simulink model "VDCv2mk2"  (R2023b)
settings: Solver=FixedStepAuto  StartTime=0.0  StopTime=10.0  RelTol=1e-3
libraries: simulink x3
(part 2 of 2)

== system VDCv2mk2/SAFETY BLOCK/APPS_IMPLAUSIBILITY/Imp ==
  Action Port : ActionPort  ActionPortLabel=if(u1 > 0.1)
  Add : Sum
  Constant : Constant  OutDataTypeStr=boolean
  Data Store Read : DataStoreRead  DataStoreName=ERROR_Counter  IndexOptions=Index vector (dialog)  Indices=1  OutputSizes=1
  Out1 : Outport  VectorParamsAs1DForOutWhenUnconnected=off
  wires:
  Data Store Read/1 -> Add/1
  Constant/1 -> Add/2
  Add/1 -> Out1/1

== system VDCv2mk2/SAFETY BLOCK/APPS_IMPLAUSIBILITY/Not Imp ==
  Action Port : ActionPort  ActionPortLabel=else
  Constant : Constant  Value=0  OutDataTypeStr=double
  0 : Outport  VectorParamsAs1DForOutWhenUnconnected=off
  wires:
  Constant/1 -> 0/1  "Boolean"

== system VDCv2mk2/SAFETY BLOCK/APPS_IMPLAUSIBILITY/Signal_Failure ==
  Action Port : ActionPort  ActionPortLabel=if(u1>u2)
  Constant : Constant
  Out1 : Outport  VectorParamsAs1DForOutWhenUnconnected=off
  wires:
  Constant/1 -> Out1/1

== system VDCv2mk2/SAFETY BLOCK/APPS_IMPLAUSIBILITY/Signal_OK ==
  Action Port : ActionPort  ActionPortLabel=else
  Constant : Constant  Value=0
  Out1 : Outport  VectorParamsAs1DForOutWhenUnconnected=off
  wires:
  Constant/1 -> Out1/1

== system VDCv2mk2/Accumulator Power/PowerLimitDetection/OK_OrLatch/Latched Error ==
  Action Port : ActionPort  ActionPortLabel=if((u1>0))
  Constant : Constant
  "Out " : Outport  VectorParamsAs1DForOutWhenUnconnected=off
  wires:
  Constant/1 -> "Out "/1

== system VDCv2mk2/Accumulator Power/PowerLimitDetection/OK_OrLatch/OK ==
  Action Port : ActionPort  ActionPortLabel=else
  Constant : Constant  Value=0
  "Out " : Outport  VectorParamsAs1DForOutWhenUnconnected=off
  wires:
  Constant/1 -> "Out "/1

== matlab function VDCv2mk2/Brake_Light ==
  data: BP input; RM input; BL output; PS input; BL_threshold input
function BL = Brake_Light(BP, RM, PS, BL_threshold)
% PS = 0 -> braking
% PS = 1 -> lift
% PS = 2 -> accelerating
% BL_threshold -> BrakePedal percentage to activate BrakeLight
    if ((RM == 5 && PS == 0) || (RM ~= 5 && BP > BL_threshold))
        BL = 1;
        return;
    else
        BL = 0;
        return;
    end
end

== matlab function VDCv2mk2/ACCELERATION/RIGIDAXLE/Rigid Axle 2024  ==
  data: Throttle_Torque input; Motor_Torque_RR output; Motor_Torque_RL output
function [Motor_Torque_RR, Motor_Torque_RL] = RigidAxle_2024(Throttle_Torque)
    
    Motor_Torque_RR = Throttle_Torque;
    Motor_Torque_RL = Throttle_Torque;

end

== matlab function VDCv2mk2/ACCELERATION/RIGIDAXLE WITH TC/Rigid Axle with TC 2024  ==
  data: MAX_SLR input; Throttle_Torque input; Motor_Torque_RR output; Motor_Torque_RL output; el_Vel_X input; Max_Vel_ms_Wheel input
function [Motor_Torque_RR, Motor_Torque_RL] = RigidAxle_TC_2024(MAX_SLR, Throttle_Torque, el_Vel_X, Max_Vel_ms_Wheel)
if (el_Vel_X < 3 || Vel_ms_wheel_RR < 3 || Vel_ms_wheel_RL < 3)
    Motor_Torque_RR = Throttle_Torque_R;
    Motor_Torque_RL = Throttle_Torque_L;
    return;
else
    persistent correction
    if isempty(correction)
        correction = 0;
    end
% SLIP RATIO CALCULATIONS
    % calculate slip ratio
    if(el_Vel_X == 0 ||Max_Vel_ms_Wheel == 0)
        SLR = 1;
    else
    SLR = (Max_Vel_ms_Wheel / el_Vel_X);
    end
% CHECK FOR EXCESIVE SLIPPING
    % SLIP RATIO LESSER THAN MAXIMUM SLIP RATIO => apply max torque times throttle factor
        if(SLR < MAX_SLR)
            Motor_Torque_RR = Throttle_Torque; 
            Motor_Torque_RL = Throttle_Torque;
            correction = 0; %set correction to 0 as tyre is not slipping
            return;
        else
        % TYRE SLIPPING => TC INTERVENES
            % LOOK FOR THE PREVIOUS CORRECTION [Nm]
            if (correction == 0) % NOT SLIPPING PREVIOUSLY
                correction = 1; % [INTERVAL TO BE DETERMINED] set the correction to the torque we want to substract
                Motor_Torque_RR = Throttle_Torque - (1/33*correction^2+1/33*correction); % substract the correction from the torque to apply
                Motor_Torque_RL = Throttle_Torque - (1/33*correction^2+1/33*correction);
                return;
            else % TYRE SLIPPING PREVIOUSLY
                correction = correction + 1; % [INTERVAL TO BE DETERMINED] set the correction to the torque we want to substract + previous corrections
                Motor_Torque_RR = Throttle_Torque - (1/33*correction^2+1/33*correction); % substract the correction from the torque to apply
                Motor_Torque_RL = Throttle_Torque - (1/33*correction^2+1/33*correction);
                return;
            end
        end
end
end

== matlab function VDCv2mk2/ENDURANCE/RIGIDAXLE WITH TC/Rigid Axle with TC 2024  ==
  data: MAX_SLR input; Throttle_Torque input; Motor_Torque_RR output; Motor_Torque_RL output; el_Vel_X input; Max_Vel_ms_Wheel input
function [Motor_Torque_RR, Motor_Torque_RL] = RigidAxle_TC_2024(MAX_SLR, Throttle_Torque, el_Vel_X, Max_Vel_ms_Wheel)
if (el_Vel_X < 3 || Vel_ms_wheel_RR < 3 || Vel_ms_wheel_RL < 3)
    Motor_Torque_RR = Throttle_Torque_R;
    Motor_Torque_RL = Throttle_Torque_L;
    return;
else
    persistent correction
    if isempty(correction)
        correction = 0;
    end
% SLIP RATIO CALCULATIONS
    % calculate slip ratio
    if(el_Vel_X == 0 ||Max_Vel_ms_Wheel == 0)
        SLR = 1;
    else
    SLR = (Max_Vel_ms_Wheel / el_Vel_X);
    end
% CHECK FOR EXCESIVE SLIPPING
    % SLIP RATIO LESSER THAN MAXIMUM SLIP RATIO => apply max torque times throttle factor
        if(SLR < MAX_SLR)
            Motor_Torque_RR = Throttle_Torque; 
            Motor_Torque_RL = Throttle_Torque;
            correction = 0; %set correction to 0 as tyre is not slipping
            return;
        else
        % TYRE SLIPPING => TC INTERVENES
            % LOOK FOR THE PREVIOUS CORRECTION [Nm]
            if (correction == 0) % NOT SLIPPING PREVIOUSLY
                correction = 1; % [INTERVAL TO BE DETERMINED] set the correction to the torque we want to substract
                Motor_Torque_RR = Throttle_Torque - (1/33*correction^2+1/33*correction); % substract the correction from the torque to apply
                Motor_Torque_RL = Throttle_Torque - (1/33*correction^2+1/33*correction);
                return;
            else % TYRE SLIPPING PREVIOUSLY
                correction = correction + 1; % [INTERVAL TO BE DETERMINED] set the correction to the torque we want to substract + previous corrections
                Motor_Torque_RR = Throttle_Torque - (1/33*correction^2+1/33*correction); % substract the correction from the torque to apply
                Motor_Torque_RL = Throttle_Torque - (1/33*correction^2+1/33*correction);
                return;
            end
        end
end
end

== matlab function VDCv2mk2/ENDURANCE/TC+TV/MATLAB Function ==
  data: steering_max_angle input; Torque_R_Nm output; Torque_L_Nm output; steering input; steering_deadzone input; Throttle_Torque input; regen_en input; cg_slip input
function [Torque_R_Nm, Torque_L_Nm] = TV(steering_max_angle, steering, steering_deadzone, Throttle_Torque, regen_en, cg_slip)

if abs(steering) <= steering_deadzone % add steering deadzone (º)
    Torque_L_Nm = Throttle_Torque;
    Torque_R_Nm = Throttle_Torque;
    return;
end
if(abs(cg_slip) > (6*pi/180)) % check for driver correcting oversteer to avoid overcorrecting
     Torque_L_Nm = Throttle_Torque;
     Torque_R_Nm = Throttle_Torque;
     return;
end
d = (abs(steering) - steering_deadzone)/(steering_max_angle - steering_deadzone) * Throttle_Torque; %evaluate delta torque for given steering angle

if regen_en == 0 && d > Throttle_Torque
     d = Throttle_Torque; %force torque to be positive to avoid balance issues
end
if steering < -steering_deadzone %if steering left, apply full torque to the emotor on the outside
       %and substract the delta from the inside one
    Torque_L_Nm = Throttle_Torque-d;
    Torque_R_Nm = Throttle_Torque;
    return;
else
%opposite case
Torque_L_Nm = Throttle_Torque;
Torque_R_Nm = Throttle_Torque-d;
return;
end
end

== matlab function VDCv2mk2/ENDURANCE/TC+TV/TC 2024 ==
  data: MAX_SLR input; Throttle_Torque_R input; Throttle_Torque_L input; Motor_Torque_RR output; Motor_Torque_RL output; el_Vel_X input; Vel_ms_wheel_RR input; Vel_ms_wheel_RL input
function [Motor_Torque_RR, Motor_Torque_RL] = TC_2024(MAX_SLR,Throttle_Torque_R, Throttle_Torque_L, el_Vel_X, Vel_ms_wheel_RR, Vel_ms_wheel_RL)
if (el_Vel_X < 3 || Vel_ms_wheel_RR < 3 || Vel_ms_wheel_RL < 3)
    Motor_Torque_RR = Throttle_Torque_R;
    Motor_Torque_RL = Throttle_Torque_L;
    return;
else
    persistent correction
    if isempty(correction)
        correction = 0;
    end

% SLIP RATIO CALCULATIONS
    % calculate slip ratio
    if(el_Vel_X == 0 || Vel_ms_wheel_RR == 0)
        SLR_RR = 1;
    else
    SLR_RR = (Vel_ms_wheel_RR / el_Vel_X);
    end
    if(el_Vel_X == 0 || Vel_ms_wheel_RL == 0)
        SLR_RL = 1;
    else
    SLR_RL = (Vel_ms_wheel_RL / el_Vel_X);
    end


% SLIP RATIO CALCULATIONS
    % calculate slip ratio
    SLR = max(SLR_RR, SLR_RL);

% CHECK FOR EXCESIVE SLIPPING
    % SLIP RATIO LESSER THAN MAXIMUM SLIP RATIO => apply max torque times throttle factor
        if(SLR < MAX_SLR)
            Motor_Torque_RR = Throttle_Torque_R; 
            Motor_Torque_RL = Throttle_Torque_L;
            correction = 0; %set correction to 0 as tyre is not slipping
            return;
        else
        % TYRE SLIPPING => TC INTERVENES
            % LOOK FOR THE PREVIOUS CORRECTION [Nm]
            if (correction == 0) % NOT SLIPPING PREVIOUSLY
                correction = 1; % [INTERVAL TO BE DETERMINED] set the correction to the torque we want to substract
                Motor_Torque_RR = Throttle_Torque_R - (1/33*correction^2+1/33*correction); % substract the correction from the torque to apply
                Motor_Torque_RL = Throttle_Torque_L - (1/33*correction^2+1/33*correction);
                return;
            else % TYRE SLIPPING PREVIOUSLY
                correction = correction + 1; % [INTERVAL TO BE DETERMINED] set the correction to the torque we want to substract + previous corrections
                Motor_Torque_RR = Throttle_Torque_R - (1/33*correction^2+1/33*correction); % substract the correction from the torque to apply
                Motor_Torque_RL = Throttle_Torque_L - (1/33*correction^2+1/33*correction);
                return;
            end
        end
end
end

== matlab function VDCv2mk2/ACCELERATION/Torque demanded by the driver ==
  data: Throttle_Torque output; AP input; pedal_sat_down input; pedal_sat_up input; max_torque input
function Throttle_Torque  = TT(AP, pedal_sat_down, pedal_sat_up, max_torque)
    if AP <= pedal_sat_down %establish the lower deadzone for the throttle pedal
        Throttle_Response = 0;

    elseif AP >= pedal_sat_up %establish the higher deadzone for the throttle pedal
        Throttle_Response = 1;

    else
        Throttle_Response = ((AP - pedal_sat_down) / (pedal_sat_up - pedal_sat_down)); %evaluate for given input
    end
    Throttle_Torque = Throttle_Response * max_torque; % set torque to max output times pedal factor
end

== matlab function VDCv2mk2/ENDURANCE/Torque/state ==
  data: AP input; AP_sat_down input; state output; AP_sat_mid input
function state = Pedal_State(AP, AP_sat_down, AP_sat_mid)
% state = 0 -> braking
% state = 1 -> lift
% state = 2 -> accelerating
state = 1;
if AP < AP_sat_down
    state = 0;
    return;
end
if AP >= AP_sat_down && AP <= AP_sat_mid
    state = 1;
    return;
end
if AP > AP_sat_mid
    state = 2;
    return;
end
end

== matlab function VDCv2mk2/AUTOX1/TC+TV/Rigid Axle with TC 2024  ==
  data: MAX_SLR input; Throttle_Torque_R input; Throttle_Torque_L input; Motor_Torque_RR output; Motor_Torque_RL output; el_Vel_X input; Vel_ms_wheel_RR input; Vel_ms_wheel_RL input
function [Motor_Torque_RR, Motor_Torque_RL] = TC_2024(MAX_SLR,Throttle_Torque_R, Throttle_Torque_L, el_Vel_X, Vel_ms_wheel_RR, Vel_ms_wheel_RL)
if (el_Vel_X < 3 || Vel_ms_wheel_RR < 3 || Vel_ms_wheel_RL < 3)
    Motor_Torque_RR = Throttle_Torque_R;
    Motor_Torque_RL = Throttle_Torque_L;
    return;
else
    persistent correction
    if isempty(correction)
        correction = 0;
    end

% SLIP RATIO CALCULATIONS
    % calculate slip ratio
    if(el_Vel_X == 0 || Vel_ms_wheel_RR == 0)
        SLR_RR = 1;
    else
    SLR_RR = (Vel_ms_wheel_RR / el_Vel_X);
    end
    if(el_Vel_X == 0 || Vel_ms_wheel_RL == 0)
        SLR_RL = 1;
    else
    SLR_RL = (Vel_ms_wheel_RL / el_Vel_X);
    end


% SLIP RATIO CALCULATIONS
    % calculate slip ratio
    SLR = max(SLR_RR, SLR_RL);

% CHECK FOR EXCESIVE SLIPPING
    % SLIP RATIO LESSER THAN MAXIMUM SLIP RATIO => apply max torque times throttle factor
        if(SLR < MAX_SLR)
            Motor_Torque_RR = Throttle_Torque_R; 
            Motor_Torque_RL = Throttle_Torque_L;
            correction = 0; %set correction to 0 as tyre is not slipping
            return;
        else
        % TYRE SLIPPING => TC INTERVENES
            % LOOK FOR THE PREVIOUS CORRECTION [Nm]
            if (correction == 0) % NOT SLIPPING PREVIOUSLY
                correction = 1; % [INTERVAL TO BE DETERMINED] set the correction to the torque we want to substract
                Motor_Torque_RR = Throttle_Torque_R - (1/33*correction^2+1/33*correction); % substract the correction from the torque to apply
                Motor_Torque_RL = Throttle_Torque_L - (1/33*correction^2+1/33*correction);
                return;
            else % TYRE SLIPPING PREVIOUSLY
                correction = correction + 1; % [INTERVAL TO BE DETERMINED] set the correction to the torque we want to substract + previous corrections
                Motor_Torque_RR = Throttle_Torque_R - (1/33*correction^2+1/33*correction); % substract the correction from the torque to apply
                Motor_Torque_RL = Throttle_Torque_L - (1/33*correction^2+1/33*correction);
                return;
            end
        end
end
end

== matlab function VDCv2mk2/SKIDPAD/TV with TC OFF /MATLAB Function ==
  data: steering_max_angle input; Torque_R_Nm output; Torque_L_Nm output; steering input; steering_deadzone input; Throttle_Torque input
function [Torque_R_Nm, Torque_L_Nm] = TV(steering_max_angle, steering, steering_deadzone, Throttle_Torque)

if abs(steering) <= steering_deadzone % add steering deadzone (º)
    Torque_L_Nm = Throttle_Torque;
    Torque_R_Nm = Throttle_Torque;
    return;
end
d = (abs(steering) - steering_deadzone)/(steering_max_angle - steering_deadzone) * Throttle_Torque; %evaluate delta torque for given steering angle
if d > Throttle_Torque
     d = Throttle_Torque; %force torque to be positive to avoid balance issues
end
if steering < -steering_deadzone %if steering left, apply full torque to the emotor on the outside
       %and substract the delta from the inside one
    Torque_L_Nm = Throttle_Torque-d;
    Torque_R_Nm = Throttle_Torque;
    return;
else
%opposite case
Torque_L_Nm = Throttle_Torque;
Torque_R_Nm = Throttle_Torque-d;
return;
end
end

== matlab function VDCv2mk2/WORKSHOP/Torque demanded by the driver ==
  data: Throttle_Torque output; AP input; pedal_sat_down input; pedal_sat_up input; max_torque input
function Throttle_Torque  = TT(AP, pedal_sat_down, pedal_sat_up, max_torque)
max_torque = max_torque / 5;
    if AP <= pedal_sat_down %establish the lower deadzone for the throttle pedal
        Throttle_Response = 0;

    elseif AP >= pedal_sat_up %establish the higher deadzone for the throttle pedal
        Throttle_Response = 1;

    else
        Throttle_Response = ((AP - pedal_sat_down) / (pedal_sat_up - pedal_sat_down)); %evaluate for given input
    end
    Throttle_Torque = Throttle_Response * max_torque; % set torque to max output times pedal factor
end

== matlab function VDCv2mk2/ENDURANCE/Torque/enable regen ==
  data: regen_en output; SOC input; max_SOC input; current input; voltage input; W_RR input; W_RL input; max_regen_torque_RR output; max_regen_torque_RL output
function [regen_en, max_regen_torque_RR, max_regen_torque_RL] = regen(SOC, max_SOC, current, voltage, W_RR, W_RL)
    max_regen_torque_RR = 0;
    max_regen_torque_RL = 0;
    regen_en = 0;
    if SOC < max_SOC
        regen_en = 1;
    end
    if SOC >= max_SOC
        regen_en = 0;
    end
    if regen_en == 1
        max_regen_torque_RR = min(current*voltage/W_RR, 27);
        max_regen_torque_RL = min(current*voltage/W_RL, 27);
    end
end

== matlab function VDCv2mk2/ENDURANCE/Torque/Torque demanded by the driver ==
  data: max_regen_torque input; regen_en input; state input; AP input; AP_sat_down input; AP_sat_mid input; tq_RR output; tq_RL output; max_torque input
function [tq_RR, tq_RL] = torque(max_regen_torque, regen_en, state, AP, AP_sat_down, AP_sat_mid, max_torque)
% state = 0 -> braking
% state = 1 -> lift
% state = 2 -> accelerating
    tq_RR = 0;
    tq_RL = 0;
    if state == 0
        if regen_en == 1
        tq_RR = -max_regen_torque * (AP  / AP_sat_down);
        tq_RL = tq_RR;
        else
            tq_RR = 0;
            tq_RL = 0;
        end
    end
    if state == 1
        tq_RR = 0;
        tq_RL = 0;
    end
    if state == 2
        tq_RR = max_torque * (AP  / (1 - AP_sat_mid));
        tq_RL = tq_RR;
    end
end

== matlab function VDCv2mk2/ENDURANCE/RIGIDAXLE/Rigid Axle 2024  ==
  data: Throttle_Torque input; Motor_Torque_RR output; Motor_Torque_RL output
function [Motor_Torque_RR, Motor_Torque_RL] = RigidAxle_2024(Throttle_Torque)
    
    Motor_Torque_RR = Throttle_Torque;
    Motor_Torque_RL = Throttle_Torque;

end

== matlab function VDCv2mk2/SKIDPAD/RIGIDAXLE/Rigid Axle 2024  ==
  data: Throttle_Torque input; Motor_Torque_RR output; Motor_Torque_RL output
function [Motor_Torque_RR, Motor_Torque_RL] = RigidAxle_2024(Throttle_Torque)
    
    Motor_Torque_RR = Throttle_Torque;
    Motor_Torque_RL = Throttle_Torque;

end

== matlab function VDCv2mk2/AUTOX1/RIGIDAXLE/Rigid Axle 2024  ==
  data: Throttle_Torque input; Motor_Torque_RR output; Motor_Torque_RL output
function [Motor_Torque_RR, Motor_Torque_RL] = RigidAxle_2024(Throttle_Torque)
    
    Motor_Torque_RR = Throttle_Torque;
    Motor_Torque_RL = Throttle_Torque;

end

== matlab function VDCv2mk2/AUTOX1/RIGIDAXLE WITH TC/Rigid Axle with TC 2024  ==
  data: MAX_SLR input; Throttle_Torque input; Motor_Torque_RR output; Motor_Torque_RL output; el_Vel_X input; Max_Vel_ms_Wheel input
function [Motor_Torque_RR, Motor_Torque_RL] = RigidAxle_TC_2024(MAX_SLR, Throttle_Torque, el_Vel_X, Max_Vel_ms_Wheel)
if (el_Vel_X < 3 || Vel_ms_wheel_RR < 3 || Vel_ms_wheel_RL < 3)
    Motor_Torque_RR = Throttle_Torque_R;
    Motor_Torque_RL = Throttle_Torque_L;
    return;
else
    persistent correction
    if isempty(correction)
        correction = 0;
    end
% SLIP RATIO CALCULATIONS
    % calculate slip ratio
    if(el_Vel_X == 0 ||Max_Vel_ms_Wheel == 0)
        SLR = 1;
    else
    SLR = (Max_Vel_ms_Wheel / el_Vel_X);
    end
% CHECK FOR EXCESIVE SLIPPING
    % SLIP RATIO LESSER THAN MAXIMUM SLIP RATIO => apply max torque times throttle factor
        if(SLR < MAX_SLR)
            Motor_Torque_RR = Throttle_Torque; 
            Motor_Torque_RL = Throttle_Torque;
            correction = 0; %set correction to 0 as tyre is not slipping
            return;
        else
        % TYRE SLIPPING => TC INTERVENES
            % LOOK FOR THE PREVIOUS CORRECTION [Nm]
            if (correction == 0) % NOT SLIPPING PREVIOUSLY
                correction = 1; % [INTERVAL TO BE DETERMINED] set the correction to the torque we want to substract
                Motor_Torque_RR = Throttle_Torque - (1/33*correction^2+1/33*correction); % substract the correction from the torque to apply
                Motor_Torque_RL = Throttle_Torque - (1/33*correction^2+1/33*correction);
                return;
            else % TYRE SLIPPING PREVIOUSLY
                correction = correction + 1; % [INTERVAL TO BE DETERMINED] set the correction to the torque we want to substract + previous corrections
                Motor_Torque_RR = Throttle_Torque - (1/33*correction^2+1/33*correction); % substract the correction from the torque to apply
                Motor_Torque_RL = Throttle_Torque - (1/33*correction^2+1/33*correction);
                return;
            end
        end
end
end

== matlab function VDCv2mk2/SKIDPAD/TC+TV/MATLAB Function ==
  data: steering_max_angle input; Torque_R_Nm output; Torque_L_Nm output; steering input; steering_deadzone input; Throttle_Torque input; cg_slip input
function [Torque_R_Nm, Torque_L_Nm] = TV(steering_max_angle, steering, steering_deadzone, Throttle_Torque, cg_slip)

if abs(steering) <= steering_deadzone % add steering deadzone (º)
    Torque_L_Nm = Throttle_Torque;
    Torque_R_Nm = Throttle_Torque;
    return;
end
if(abs(cg_slip) > (6*pi/180)) % check for driver correcting oversteer to avoid overcorrecting
     Torque_L_Nm = Throttle_Torque;
     Torque_R_Nm = Throttle_Torque;
     return;
end
d = (abs(steering) - steering_deadzone)/(steering_max_angle - steering_deadzone) * Throttle_Torque; %evaluate delta torque for given steering angle
if d > Throttle_Torque
     d = Throttle_Torque; %force torque to be positive to avoid balance issues
end
if steering < -steering_deadzone %if steering left, apply full torque to the emotor on the outside
       %and substract the delta from the inside one
    Torque_L_Nm = Throttle_Torque-d;
    Torque_R_Nm = Throttle_Torque;
    return;
else
%opposite case
Torque_L_Nm = Throttle_Torque;
Torque_R_Nm = Throttle_Torque-d;
return;
end
end

== matlab function VDCv2mk2/SKIDPAD/TC+TV/Rigid Axle with TC 2024  ==
  data: MAX_SLR input; Throttle_Torque_R input; Throttle_Torque_L input; Motor_Torque_RR output; Motor_Torque_RL output; el_Vel_X input; Vel_ms_wheel_RR input; Vel_ms_wheel_RL input
function [Motor_Torque_RR, Motor_Torque_RL] = TC_2024(MAX_SLR,Throttle_Torque_R, Throttle_Torque_L, el_Vel_X, Vel_ms_wheel_RR, Vel_ms_wheel_RL)
if (el_Vel_X < 3 || Vel_ms_wheel_RR < 3 || Vel_ms_wheel_RL < 3)
    Motor_Torque_RR = Throttle_Torque_R;
    Motor_Torque_RL = Throttle_Torque_L;
    return;
else
    persistent correction
    if isempty(correction)
        correction = 0;
    end

% SLIP RATIO CALCULATIONS
    % calculate slip ratio
    if(el_Vel_X == 0 || Vel_ms_wheel_RR == 0)
        SLR_RR = 1;
    else
    SLR_RR = (Vel_ms_wheel_RR / el_Vel_X);
    end
    if(el_Vel_X == 0 || Vel_ms_wheel_RL == 0)
        SLR_RL = 1;
    else
    SLR_RL = (Vel_ms_wheel_RL / el_Vel_X);
    end


% SLIP RATIO CALCULATIONS
    % calculate slip ratio
    SLR = max(SLR_RR, SLR_RL);

% CHECK FOR EXCESIVE SLIPPING
    % SLIP RATIO LESSER THAN MAXIMUM SLIP RATIO => apply max torque times throttle factor
        if(SLR < MAX_SLR)
            Motor_Torque_RR = Throttle_Torque_R; 
            Motor_Torque_RL = Throttle_Torque_L;
            correction = 0; %set correction to 0 as tyre is not slipping
            return;
        else
        % TYRE SLIPPING => TC INTERVENES
            % LOOK FOR THE PREVIOUS CORRECTION [Nm]
            if (correction == 0) % NOT SLIPPING PREVIOUSLY
                correction = 1; % [INTERVAL TO BE DETERMINED] set the correction to the torque we want to substract
                Motor_Torque_RR = Throttle_Torque_R - (1/33*correction^2+1/33*correction); % substract the correction from the torque to apply
                Motor_Torque_RL = Throttle_Torque_L - (1/33*correction^2+1/33*correction);
                return;
            else % TYRE SLIPPING PREVIOUSLY
                correction = correction + 1; % [INTERVAL TO BE DETERMINED] set the correction to the torque we want to substract + previous corrections
                Motor_Torque_RR = Throttle_Torque_R - (1/33*correction^2+1/33*correction); % substract the correction from the torque to apply
                Motor_Torque_RL = Throttle_Torque_L - (1/33*correction^2+1/33*correction);
                return;
            end
        end
end
end

== matlab function VDCv2mk2/AUTOX1/TC+TV/MATLAB Function ==
  data: steering_max_angle input; Torque_R_Nm output; Torque_L_Nm output; steering input; steering_deadzone input; Throttle_Torque input
function [Torque_R_Nm, Torque_L_Nm] = TV(steering_max_angle, steering, steering_deadzone, Throttle_Torque)
    if abs(steering) <= steering_deadzone % add steering deadzone (º)
        Torque_L_Nm = Throttle_Torque;
        Torque_R_Nm = Throttle_Torque;
        return;
    end
        d = (abs(steering) - steering_deadzone)/(steering_max_angle - steering_deadzone) * Throttle_Torque; %evaluate delta torque for given steering angle
    if d > Throttle_Torque
         d = Throttle_Torque; %force torque to be positive to avoid balance issues
    end
    if steering < -steering_deadzone %if steering left, apply more torque to the outer wheel
        Torque_L_Nm = Throttle_Torque;
        Torque_R_Nm = Throttle_Torque+d;
        return;
    else
        %opposite case
        Torque_L_Nm = Throttle_Torque+d;
        Torque_R_Nm = Throttle_Torque;
        return;
    end
end

== matlab function VDCv2mk2/SKIDPAD/Torque demanded by the driver ==
  data: Throttle_Torque output; AP input; pedal_sat_down input; pedal_sat_up input; max_torque input
function Throttle_Torque  = TT(AP, pedal_sat_down, pedal_sat_up, max_torque)
    if AP <= pedal_sat_down %establish the lower deadzone for the throttle pedal
        Throttle_Response = 0;

    elseif AP >= pedal_sat_up %establish the higher deadzone for the throttle pedal
        Throttle_Response = 1;

    else
        Throttle_Response = ((AP - pedal_sat_down) / (pedal_sat_up - pedal_sat_down)); %evaluate for given input
    end
    Throttle_Torque = Throttle_Response * max_torque; % set torque to max output times pedal factor
end

== matlab function VDCv2mk2/AUTOX1/Torque demanded by the driver ==
  data: Throttle_Torque output; AP input; pedal_sat_down input; pedal_sat_up input; max_torque input
function Throttle_Torque  = TT(AP, pedal_sat_down, pedal_sat_up, max_torque)
    if AP <= pedal_sat_down %establish the lower deadzone for the throttle pedal
        Throttle_Response = 0;

    elseif AP >= pedal_sat_up %establish the higher deadzone for the throttle pedal
        Throttle_Response = 1;

    else
        Throttle_Response = ((AP - pedal_sat_down) / (pedal_sat_up - pedal_sat_down)); %evaluate for given input
    end
    Throttle_Torque = Throttle_Response * max_torque; % set torque to max output times pedal factor
end
